simulink model "delay_force_pos"  (R2020b)
settings: Solver=ode45  StartTime=0.0  StopTime=10  FixedStep=Ts  MinStep=1e-5  RelTol=1e-5
undefined symbols (not defined in the file): A_int, b, Be, Bh_i, Bs, delayT, Dh, DiscIntNeverNeededParam, Dm, Ds, Fc, Fip, Jh_i, Ke, Kh, Kh_i, Ks, Mm, Ms, Ts, xe
libraries: simulink x1, cstblocks x1
settings Model: Creator=simon  LastModifiedBy=simon
settings SolverCC: AlgebraicLoopSolver=LineSearch

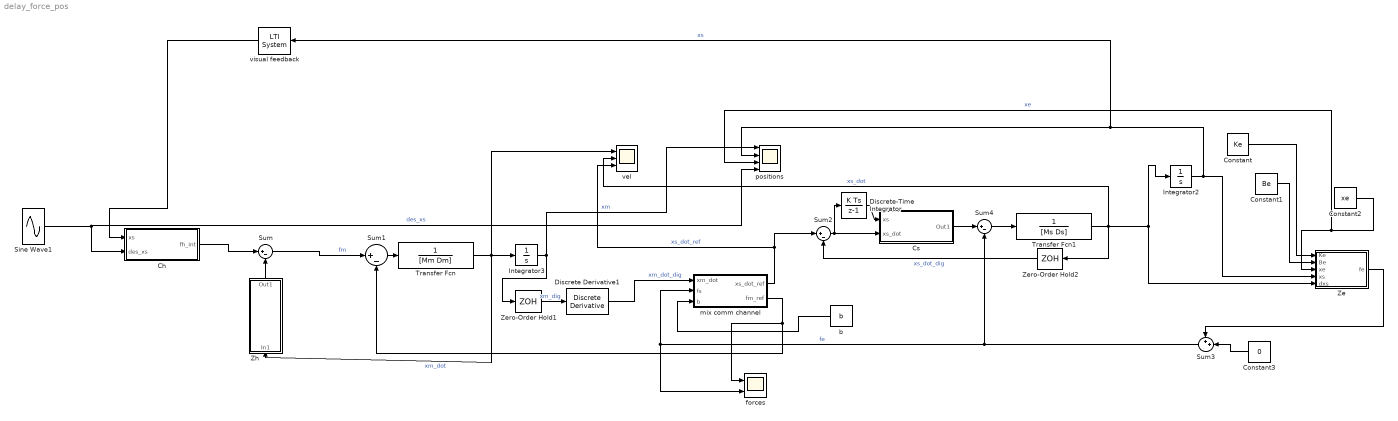
== system delay_force_pos ==
  Ch : Subsystem
  Constant : Constant  Value=Ke
  Constant1 : Constant  Value=Be
  Constant2 : Constant  Value=xe
  Constant3 : Constant  Value=0
  Cs : Subsystem
  Discrete Derivative1 : simulink/Discrete/Discrete Derivative  gainval=1.0  ICPrevScaledInput=0.0  OutMin=[]  OutMax=[]  OutDataType=fixdt(1, 16)  OutScaling=2^-10  DoSatur=off
  Discrete-Time Integrator : DiscreteIntegrator  SampleTime=-1  ICPrevOutput=DiscIntNeverNeededParam  ICPrevScaledInput=DiscIntNeverNeededParam
  Integrator2 : Integrator
  Integrator3 : Integrator
  Sine Wave1 : Sin  Amplitude=A_int  Frequency=2*pi*Fc  SampleTime=0
  Sum{,1..2,4} (4 alike) : Sum  Inputs=|+-
  Sum3 : Sum  Inputs=++|
  Transfer Fcn : TransferFcn  Denominator=[Mm Dm]
  Transfer Fcn1 : TransferFcn  Denominator=[Ms Ds]
  Ze : MATLAB Function  TreatAsAtomicUnit=on
  Zero-Order Hold1 : ZeroOrderHold  SampleTime=Ts
  Zero-Order Hold2 : ZeroOrderHold  SampleTime=Ts
  Zh : Subsystem
  b : Constant  Value=b
  forces : Scope  NumInputPorts=2
  mix comm channel : Subsystem
  positions : Scope  NumInputPorts=4
  vel : Scope  NumInputPorts=3
  visual feedback : cstblocks/LTI System  sys=1  IC=[]
  wires:
  Zh/1(Out1) -> Sum/2
  Sum1/1 -> Transfer Fcn/1
  Sum4/1 -> Transfer Fcn1/1
  Transfer Fcn1/1 -> vel/2, Integrator2/1, Ze/5(dxs), Zero-Order Hold2/1  "xs_dot"
  Ze/1(fe) -> Sum3/1
  Integrator2/1 -> visual feedback/1, positions/2, Ze/4(xs)  "xs"
  Constant2/1 -> positions/3, Ze/3(xe)  "xe"
  Constant1/1 -> Ze/2(Be)
  Constant/1 -> Ze/1(Ke)
  Sum/1 -> Sum1/1  "fm"
  Transfer Fcn/1 -> vel/1, Integrator3/1, Zh/1(In1)  "xm_dot"
  mix comm channel/2(fm_ref) -> forces/1, Sum1/2
  mix comm channel/1(xs_dot_ref) -> vel/3, Sum2/1  "xs_dot_ref"
  Sum2/1 -> Discrete-Time Integrator/1, Cs/2(xs_dot)
  Discrete-Time Integrator/1 -> Cs/1(xs)
  Cs/1(Out1) -> Sum4/1
  Sum3/1 -> forces/2, mix comm channel/2(fs), Sum4/2  "fe"
  Constant3/1 -> Sum3/2
  b/1 -> mix comm channel/3(b)
  Integrator3/1 -> positions/1, Zero-Order Hold1/1  "xm"
  Zero-Order Hold1/1 -> Discrete Derivative1/1  "xm_dig"
  Discrete Derivative1/1 -> mix comm channel/1(xm_dot)  "xm_dot_dig"
  Zero-Order Hold2/1 -> Sum2/2  "xs_dot_dig"
  Sine Wave1/1 -> positions/4, Ch/2(des_xs)  "des_xs"
  Ch/1(fh_int) -> Sum/1
  visual feedback/1 -> Ch/1(xs)

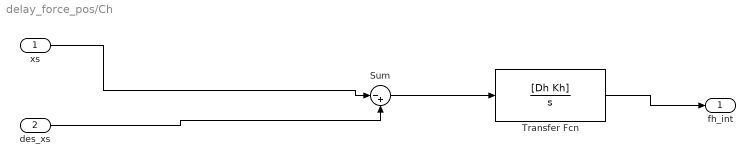
== system delay_force_pos/Ch ==
  xs : Inport
  des_xs : Inport  Port=2
  Sum : Sum  Inputs=|-+
  Transfer Fcn : TransferFcn  Numerator=[Dh Kh]  Denominator=[1 0]
  fh_int : Outport
  wires:
  xs/1 -> Sum/1
  des_xs/1 -> Sum/2
  Sum/1 -> Transfer Fcn/1
  Transfer Fcn/1 -> fh_int/1

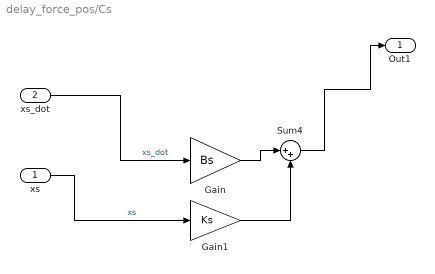
== system delay_force_pos/Cs ==
  xs : Inport
  xs_dot : Inport  Port=2
  Gain : Gain  Gain=Bs
  Gain1 : Gain  Gain=Ks
  Sum4 : Sum  Inputs=|++
  Out1 : Outport
  wires:
  Gain1/1 -> Sum4/2
  Sum4/1 -> Out1/1
  xs_dot/1 -> Gain/1  "xs_dot"
  Gain/1 -> Sum4/1
  xs/1 -> Gain1/1  "xs"

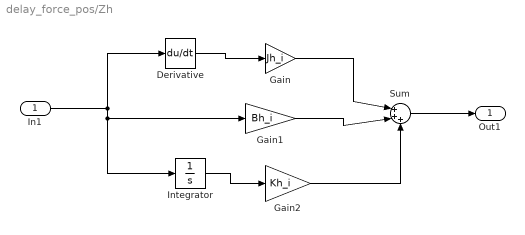
== system delay_force_pos/Zh ==
  In1 : Inport
  Derivative : Derivative
  Gain : Gain  Gain=Jh_i
  Gain1 : Gain  Gain=Bh_i
  Gain2 : Gain  Gain=Kh_i
  Integrator : Integrator
  Sum : Sum  Inputs=|+++
  Out1 : Outport
  wires:
  Derivative/1 -> Gain/1
  Integrator/1 -> Gain2/1
  In1/1 -> Integrator/1, Gain1/1, Derivative/1
  Gain/1 -> Sum/1
  Gain1/1 -> Sum/2
  Gain2/1 -> Sum/3
  Sum/1 -> Out1/1

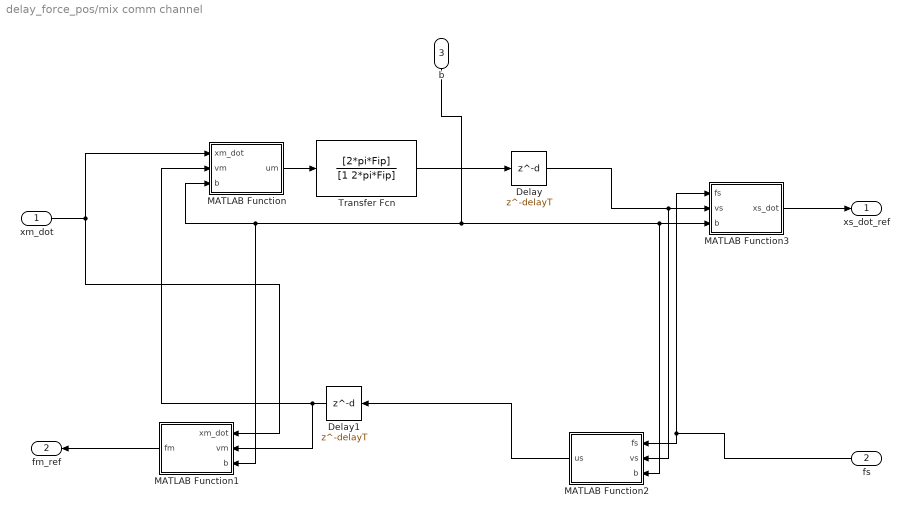
== system delay_force_pos/mix comm channel ==
  xm_dot : Inport
  fs : Inport  Port=2
  b : Inport  Port=3
  Delay : Delay  DelayLength=delayT  SampleTime=Ts
  Delay1 : Delay  DelayLength=delayT  SampleTime=Ts
  MATLAB Function : MATLAB Function  TreatAsAtomicUnit=on
  MATLAB Function1 : MATLAB Function  TreatAsAtomicUnit=on
  MATLAB Function2 : MATLAB Function  TreatAsAtomicUnit=on
  MATLAB Function3 : MATLAB Function  TreatAsAtomicUnit=on
  Transfer Fcn : TransferFcn  Numerator=[2*pi*Fip]  Denominator=[1 2*pi*Fip]
  xs_dot_ref : Outport
  fm_ref : Outport  Port=2
  wires:
  b/1 -> MATLAB Function1/3(b), MATLAB Function/3(b), MATLAB Function2/3(b), MATLAB Function3/3(b)
  xm_dot/1 -> MATLAB Function1/1(xm_dot), MATLAB Function/1(xm_dot)
  MATLAB Function1/1(fm) -> fm_ref/1
  fs/1 -> MATLAB Function3/1(fs), MATLAB Function2/1(fs)
  MATLAB Function3/1(xs_dot) -> xs_dot_ref/1
  MATLAB Function/1(um) -> Transfer Fcn/1
  Delay/1 -> MATLAB Function2/2(vs), MATLAB Function3/2(vs)
  Delay1/1 -> MATLAB Function/2(vm), MATLAB Function1/2(vm)
  Transfer Fcn/1 -> Delay/1
  MATLAB Function2/1(us) -> Delay1/1

== matlab function delay_force_pos/Ze ==
  data: Ke input; fe output; Be input; xe input; xs input; dxs input
function fe = env(Ke, Be, xe, xs, dxs)
    if xs > xe
        fe = Ke*(xs-xe)+Be*max(dxs, 0);
    else
        fe = 0;
    end

== matlab function delay_force_pos/mix comm channel/MATLAB Function ==
  data: xm_dot input; um output; vm input; b input
function um = fcn(xm_dot, vm, b)

um = sqrt(2*b)*xm_dot+vm;

== matlab function delay_force_pos/mix comm channel/MATLAB Function1 ==
  data: xm_dot input; fm output; vm input; b input
function fm = fcn(xm_dot, vm, b)

fm = b*xm_dot+sqrt(2*b)*vm;

== matlab function delay_force_pos/mix comm channel/MATLAB Function2 ==
  data: fs input; us output; vs input; b input
function us = fcn(fs, vs, b)

us = sqrt(2/b)*fs-vs;

== matlab function delay_force_pos/mix comm channel/MATLAB Function3 ==
  data: fs input; xs_dot output; vs input; b input
function xs_dot = fcn(fs, vs, b)

xs_dot = -1/b*(fs-sqrt(2*b)*vs);
